simulink model "tf_model"  (R2012b)
settings: Solver=ode45  StartTime=0.0  StopTime=Tf  MaxStep=1e-3  RelTol=1e-3
values from neighbouring files (symbols this model uses):
  den_Gpre = C_obs*inv(A_obs-B_obs*K)*B_obs    [sv__feedback__observer_driver.m]    (also in sv__feedback_driver.m = C*inv(A-B*K)*B; tf_sv_driver.m = 1)
  num_Gpre = -1    [sv__feedback__observer_driver.m]    (also in sv__feedback_driver.m; tf_sv_driver.m = 1)
undefined symbols (not defined in the file or in its folder): den_Gc, den_Gp, num_Gc, num_Gp
settings Model: Creator=student  LastModifiedBy=throne
settings DataIOCC: SignalLoggingSaveFormat=ModelDataLogs  SignalLoggingName=sigsOut
settings OptimizationCC: InitFltsAndDblsToZero=on
settings DebuggingCC: SaveWithParameterizedLinksMsg=none  SignalResolutionControl=TryResolveAllWithWarning  SolverPrmCheckMsg=none  MultiTaskDSMMsg=warning  MultiTaskCondExecSysMsg=none  FcnCallInpInsideContextMsg=UseLocalSettings  StrictBusMsg=None
settings HardwareCC: TargetUnknown=on
settings RTWCC: IncludeERTFirstTime=on
settings GRTTargetCC: CombineOutputUpdateFcns=off  GRTInterface=on

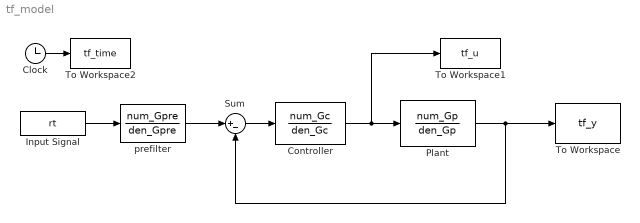
== system tf_model ==
  Clock : Clock
  Controller : TransferFcn  Numerator=num_Gc  Denominator=den_Gc
  "Input Signal " : FromWorkspace  VariableName=rt  SampleTime=0
  Plant : TransferFcn  Numerator=num_Gp  Denominator=den_Gp
  Sum : Sum  Inputs=|+-  SaturateOnIntegerOverflow=on
  To Workspace : ToWorkspace  VariableName=tf_y  SampleTime=-1
  To Workspace1 : ToWorkspace  VariableName=tf_u  SampleTime=-1
  To Workspace2 : ToWorkspace  VariableName=tf_time  SampleTime=-1
  prefilter : TransferFcn  Numerator=num_Gpre  Denominator=den_Gpre
  wires:
  Plant/1 -> Sum/2, To Workspace/1
  Sum/1 -> Controller/1
  Clock/1 -> To Workspace2/1
  prefilter/1 -> Sum/1
  "Input Signal "/1 -> prefilter/1
  Controller/1 -> To Workspace1/1, Plant/1
